simulink model "sm_excv_track1_sprocket"  (R2026a)
settings: Solver=ode23t  StopTime=15  FixedStep=2e-4  AbsTol=1e-3
StartFcn:
  | tic
StopFcn:
  | Elapsed_Sim_Time = toc;
  | disp(['Elapsed Sim Time = ' num2str(Elapsed_Sim_Time)]);
undefined symbols (not defined in the file or in its folder): Excv, X, Y, Z
libraries: sm_lib x11, fl_lib x2, nesl_utility x2, sm_trackV_lib_chain_contact_s46 x2, sm_trackV_lib_chain_underc_elem x1, simulink x1, sm_trackV_lib_chain_contact_s46r9 x1, sm_trackV_lib_chain_track_s46 x1, sm_trackV_lib_chain_underc_i1u2l7 x1
CloseFcn:
  | try,close(h1_sm_excv_track_sprocket),end
  | clear h1_sm_excv_track_sprocket
  | try,close(h2_sm_excv_track_sprocket),end
  | clear h2_sm_excv_track_sprocket
  | try,close(h3_sm_excv_track_sprocket),end
  | clear h3_sm_excv_track_sprocket
  | try,close(h4_sm_excv_track_sprocket),end
  | clear h4_sm_excv_track_sprocket
  | 
  | 
  | clear simlog_sm_excv_track_single_sprocket
  | clear logsout_sm_excv_track_single_sprocket
Description:
  | Excavator Track (Single) Hanging on Sprocket
  | Copyright 2023-2026 The MathWorks, Inc.
settings Model: Creator=evo  LastModifiedBy=smiller
settings SolverCC: ExtrapolationOrder=1.0
settings DataIOCC: SignalLoggingName=logsout_sm_excv_track1_sprocket
settings DebuggingCC: SymbolicDimsDataTypeCodeGenerationDiagnostic=none
settings SimscapeCC: SimscapeNominalValues="[{\"value\":\"1\",\"unit\":\"A\"},{\"value\":\"1\",\"unit\":\"bar\"},{\"value\":\"1\",\"unit\":\"cm^2\"},{\"value\":\"1\",\"unit\":\"cm^3/s\"},{\"value\":\"1\",\"unit\":\"kJ/kg\"},{\"value\":\"1\",\"unit\":\"kW\"},{\"value\":\"1\",\"unit\":\"l\"},{\"value\":\"1\",\"unit\":\"N\"},{\"value\":\"1\",\"unit\":\"N*m\"},{\"value\":\"1\",\"unit\":\"V\"}]"  SimscapeLogSimulationStatistics=on  SimscapeLogName=simlog_sm_excv_track1_sprocket  SimscapeLogLimitData=off
settings DiagnosticsConfigSet: SimMechanicsConflictingReferenceFrames=none
settings ExplorerConfigSet: InternalSimMechanicsExplorerSettings="<ExplorerConfiguration><canonicalview>default</canonicalview><AnimationSetting><BasePlaybackSpeed>1.0</BasePlaybackSpeed><PlaybackSpeedFactor>1.0</PlaybackSpeedFactor></AnimationSetting><TilePanel><TileInfo><Tiles Columns=\"1\" Count=\"1\" Rows=\"1\"><Column Weight=\"1\"/><Row Weight=\"1\"/><Tile Height=\"1\" Width=\"1\" X=\"0\" Y=\"0\"/></Tiles></TileInfo><SceneInfo><SceneViewer><BGColor><R>1</R><G>1</G><B>1</B></BGColor><Camera><DoPerspective>off</DoPerspective><Position><X>-8.59833966249112791e-08</X><Y>-1.5052729587084539</Y><Z>-1.88886838203652996</Z></Position><Center><X>-8.59833966249112791e-08</X><Y>1.09999994761235231</Y><Z>-1.88886838203652996</Z></Center><Up><X>0</X><Y>-0</Y><Z>1</Z></Up><ViewLimDist>1</ViewLimDist><YLim>2.41010291099548368</YLim><XLim>4.22052667248343027</XLim></Camera></SceneViewer></SceneInfo></TilePanel><MechEditorPanel><Cameras/><GfxPanelCameraMap/><VideoCreator><PlaybackSpeedRatio>1.0</PlaybackSpeedRatio><FrameRate>30</FrameRate><VideoFormat>Motion JPEG AVI</VideoFormat><FrameSize>auto</FrameSize></VideoCreator></MechEditorPanel></ExplorerConfiguration>"

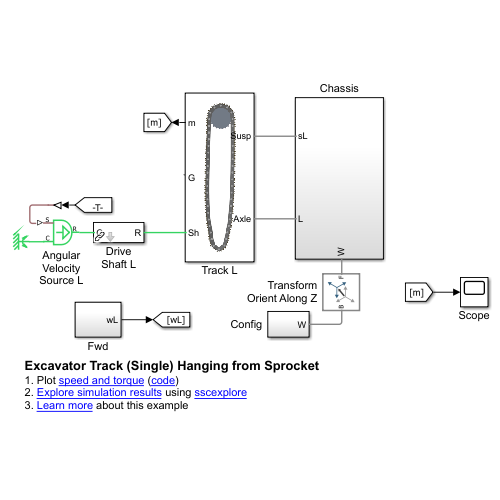
[thumbnail: Simulink's stored preview of the top-level diagram]
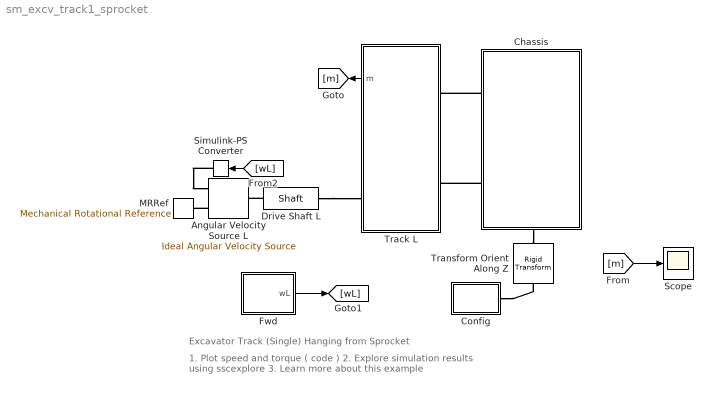
== system sm_excv_track1_sprocket ==
  note: Excavator Track (Single) Hanging from Sprocket
  note: 1. Plot speed and torque ( code )
      | 2. Explore simulation results using sscexplore
      | 3. Learn more about this example
  Angular Velocity Source L : fl_lib/Mechanical/Mechanical Sources/Ideal Angular Velocity Source
  Chassis : Subsystem
      settings: PortSchema="{\"entries\":[{\"content\":{\"sides\":[{\"content\":{\"connectorIds\":[\"LConn1\",\"LConn2\"]},\"type\":\"ConnectorPlacement.EquallySpacedRectSide\",\"uuid\":\"edd0f9cd-c75d-460e-8747-c453c06c3b51\"},{\"content\":{\"side\":\"RIGHT\"},\"type\":\"ConnectorPlacement.EquallySpacedRectSide\",\"uuid\":\"aac0b74e-f978-42e3-a6a1-4bc72aaab1ab\"},{\"content\":{\"side\":\"TOP\"},\"type\":\"ConnectorPlacement.EquallySpacedRectSide\",\"uuid\":\"f25955ca-c2f5-46fd-b059-2b680dae975d\"},{\"content\":{\"connectorIds\":[\"RConn1\"],\"side\":\"BOTTOM\"},\"type\":\"ConnectorPlacement.EquallySpacedRectSide\",\"uuid\":\"7501e828-daf5-40c9-b971-42e639c94cdf\"}]},\"type\":\"ConnectorPlacement.EquallySpacedConnector\",\"uuid\":\"6826b738-8ce7-493d-aa91-65501067c2e5\"}],\"packageUris\":[\"http://schema.mathworks.com/mf0/Connector/R2020b\"],\"version\":\"1.0\"}"
  Config : Subsystem
  Drive Shaft L : sm_trackV_lib_chain_underc_elem/Shaft  k_shaft=Excv.Drive.Shaft.k  b_shaft=Excv.Drive.Shaft.b
  Fwd : Subsystem  VariantControl=Fwd
  MRRef : fl_lib/Mechanical/Rotational Elements/Mechanical Rotational Reference
  Scope : Scope
      settings: ActiveDisplayYMinimum=-3157.84691  ActiveDisplayYMaximum=5645.58158
  Simulink-PS Converter : nesl_utility/Simulink-PS Converter  PhysicalDomain=network_engine_domain  SubClassName=ps_input  LeftPortType=input  RightPortType=output  PseudoPeriodic=off  Frequencies=[]  NoiseDistribution=none  NoiseParameters=[]  Unit=1  AffineConversion=off  FilteringAndDerivatives=provide  SimscapeFilterOrder=1  InputFilterTimeConstant=0.001  UdotUserProvided=0
  Track L : Subsystem
      settings: LibrarySourceBlock=sm_excv_lower_frame_lib/Undercarriage
      mask Display: image('sm_excv_track_sprocket_IMAGE.png');
  Transform Orient Along Z : sm_lib/Frames and Transforms/Rigid Transform  RotationMethod=StandardAxis  FollAlignAxisA=+X  BaseAlignAxisA=+Y  FollAlignAxisB=+Y  BaseAlignAxisB=+Z  RotationStandardAxis=+Y  RotationAngle=90  RotationAngleUnits=deg  RotationArbitraryAxis=[0 0 1]  RotationSequenceAxes=FollowerAxes  RotationSequence=XYX  RotationSequenceAngles=[0 0 0]  RotationSequenceAnglesUnits=deg  RotationMatrix=[1 0 0; 0 1 0; 0 0 1]  Quaternion=[1 0 0 0]  TranslationMethod=None  TranslationCartesianOffset=[0 0 0]  TranslationCartesianOffsetUnits=m  TranslationStandardAxis=+Z  TranslationStandardOffset=0  TranslationStandardOffsetUnits=m  TranslationROffset=0  TranslationROffsetUnits=m  TranslationThetaOffset=0  TranslationThetaOffsetUnits=deg  TranslationZOffset=0  TranslationZOffsetUnits=m
  wires:
  Track L/1(m) -> [m]
  [m] -> Scope/1
  [wL] -> Simulink-PS Converter/1
  Fwd/1(wL) -> [wL]
  connections:
  Chassis/RConn1 -- Transform Orient Along Z/RConn1
  Chassis/LConn2 -- Track L/LConn2
  Config/LConn1 -- Transform Orient Along Z/LConn1
  Angular Velocity Source L/RConn2 -- MRRef/LConn1
  Simulink-PS Converter/RConn1 -- Angular Velocity Source L/RConn1
  Drive Shaft L/LConn1 -- Angular Velocity Source L/LConn1
  Drive Shaft L/RConn1 -- Track L/RConn2
  Chassis/LConn1 -- Track L/LConn1

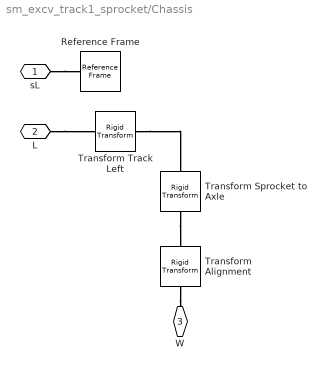
== system sm_excv_track1_sprocket/Chassis ==
  Reference Frame : sm_lib/Frames and Transforms/Reference Frame
  Transform Alignment : sm_lib/Frames and Transforms/Rigid Transform  RotationMethod=AlignedAxes  FollAlignAxisA=+X  BaseAlignAxisA=+X  FollAlignAxisB=+Y  BaseAlignAxisB=+Z  RotationStandardAxis=+Z  RotationAngle=0.0  RotationAngleUnits=deg  RotationArbitraryAxis=[0 0 1]  RotationSequenceAxes=FollowerAxes  RotationSequence=XYX  RotationSequenceAngles=[0 0 0]  RotationSequenceAnglesUnits=deg  RotationMatrix=[1 0 0; 0 1 0; 0 0 1]  Quaternion=[1 0 0 0]  TranslationMethod=None  TranslationCartesianOffset=[0 0 0]  TranslationCartesianOffsetUnits=m  TranslationStandardAxis=+Z  TranslationStandardOffset=0  TranslationStandardOffsetUnits=m  TranslationROffset=0  TranslationROffsetUnits=m  TranslationThetaOffset=0  TranslationThetaOffsetUnits=deg  TranslationZOffset=0  TranslationZOffsetUnits=m
  Transform Sprocket to Axle : sm_lib/Frames and Transforms/Rigid Transform  RotationMethod=None  FollAlignAxisA=+X  BaseAlignAxisA=+Y  FollAlignAxisB=+Y  BaseAlignAxisB=+Z  RotationStandardAxis=+Z  RotationAngle=0.0  RotationAngleUnits=deg  RotationArbitraryAxis=[0 0 1]  RotationSequenceAxes=FollowerAxes  RotationSequence=XYX  RotationSequenceAngles=[0 0 0]  RotationSequenceAnglesUnits=deg  RotationMatrix=[1 0 0; 0 1 0; 0 0 1]  Quaternion=[1 0 0 0]  TranslationMethod=Cartesian  TranslationCartesianOffset=[Excv.Frame.AxleX -Excv.Frame.AxleY 0]  TranslationCartesianOffsetUnits=m  TranslationStandardAxis=+Z  TranslationStandardOffset=0  TranslationStandardOffsetUnits=m  TranslationROffset=0  TranslationROffsetUnits=m  TranslationThetaOffset=0  TranslationThetaOffsetUnits=deg  TranslationZOffset=0  TranslationZOffsetUnits=m
  Transform Track Left : sm_lib/Frames and Transforms/Rigid Transform  RotationMethod=None  FollAlignAxisA=+X  BaseAlignAxisA=+Y  FollAlignAxisB=+Y  BaseAlignAxisB=+Z  RotationStandardAxis=+X  RotationAngle=90  RotationAngleUnits=deg  RotationArbitraryAxis=[0 0 1]  RotationSequenceAxes=FollowerAxes  RotationSequence=XYX  RotationSequenceAngles=[0 0 0]  RotationSequenceAnglesUnits=deg  RotationMatrix=[1 0 0; 0 1 0; 0 0 1]  Quaternion=[1 0 0 0]  TranslationMethod=StandardAxis  TranslationCartesianOffset=[-46.4567 43.3071 -1.4567]  TranslationCartesianOffsetUnits=m  TranslationStandardAxis=-Z  TranslationStandardOffset=1.1  TranslationStandardOffsetUnits=m  TranslationROffset=0  TranslationROffsetUnits=m  TranslationThetaOffset=0  TranslationThetaOffsetUnits=deg  TranslationZOffset=0  TranslationZOffsetUnits=m
  sL : PMIOPort  Side=Left
  L : PMIOPort  Port=2  Side=Left
  W : PMIOPort  Port=3  Side=Right
  connections:
  Transform Alignment/LConn1 -- W/RConn1
  Transform Sprocket to Axle/LConn1 -- Transform Alignment/RConn1
  L/RConn1 -- Transform Track Left/RConn1
  Transform Track Left/LConn1 -- Transform Sprocket to Axle/RConn1
  sL/RConn1 -- Reference Frame/RConn1

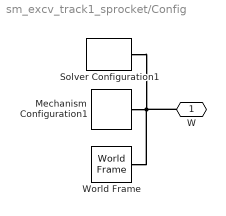
== system sm_excv_track1_sprocket/Config ==
  Mechanism Configuration1 : sm_lib/Utilities/Mechanism Configuration  UniformGravity=Constant  GravityVector=[0 0 -9.80665]  GravityVectorUnits=m/s^2  LinearizationDelta=0.001  JointModeTransitionNonlinearIterations=2
  Solver Configuration1 : nesl_utility/Solver Configuration  PhysicalDomain=network_engine_domain  SubClassName=solver  LeftPortType=input  RightPortType=generic  Tones=[]  Harmonics=[]  SimulateNoise=off  Profile=off  UseLocalSampling=off  EnableSwitchedLinearOptims=on  FrequencyDomain=off  UseCCode=off  RelTol=0.001  AbsTol=0.001  MinStep=1e-09  ToWorkspace=off  RevertToSquareIcSolve=off  NumHomotopyIterations=100  PhasorMode=off  PhasorModeNumHarmonics=1  ConsistencySolver=NEWTON_FTOL  CanonicalOrdering=UNORDERED  OptimizeIntermediates=UNOPTIMIZED  IndexReductionMethod=DerivativeReplacement  DoDC=off  ResidualTolerance=1e-09  ConsistencyTolSource=GLOBAL  ConsistencyAbsTol=0.001  ConsistencyRelTol=0.001  ConsistencyTolFactor=0.001  UseLocalSolver=off  LocalSolverChoice=NE_BACKWARD_EULER_ADVANCER  ResolveIndetEquations=on  FunctionEvalNumThread=1  LocalSolverSampleTime=0.001  DoFixedCost=off  MaxNonlinIter=3  MaxModeIter=2  ComputeImpulses=off  ImpulseIterations=2  LinearAlgebra=auto  LinearAlgebraNumThread=0  EquationFormulation=NE_TIME_EF  DelaysMemoryBudget=1024  AutomaticFiltering=on  FilteringTimeConstant=0.001  PartitionStorageMethod=AS_NEEDED  PartitionMemoryBudget=1024  PartitionMethod=ROBUST  MultibodyUseLocalSolver=off  MultibodyLocalSolverChoice=ODE1  MultibodyLocalSolverSampleTime=0.001
  World Frame : sm_lib/Frames and Transforms/World Frame
  W : PMIOPort  Side=Left
  connections:
  W/RConn1 -- Solver Configuration1/RConn1 -- Mechanism Configuration1/RConn1 -- World Frame/RConn1

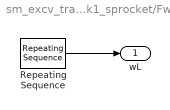
== system sm_excv_track1_sprocket/Fwd ==
  Repeating Sequence : simulink/Sources/Repeating Sequence  rep_seq_t=[0 2 2.01 40]  rep_seq_y=[0 0 3 3]
  wL : Outport
  wires:
  Repeating Sequence/1 -> wL/1

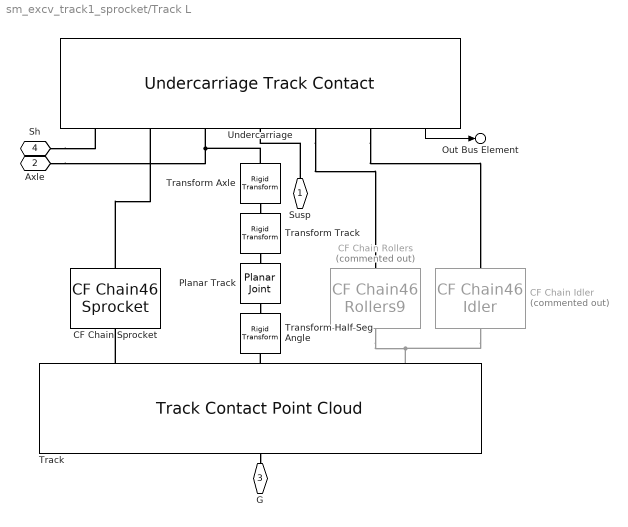
== system sm_excv_track1_sprocket/Track L ==
  CF Chain Idler : sm_trackV_lib_chain_contact_s46/CF Chain46 Idler  Commented=on  K_Idler=Excv.CFP.Idler.K  B_Idler=Excv.CFP.Idler.B  TW_Idler=Excv.CFP.Idler.TW
      settings: LibrarySourceBlock=sm_chain_drive_lib/CF_Idler_full
  CF Chain Rollers : sm_trackV_lib_chain_contact_s46r9/CF Chain46 Rollers9  Commented=on  K_Roller=Excv.Contact.Roller.K  B_Roller=Excv.Contact.Roller.B  TW_Roller=Excv.Contact.Roller.TW
      settings: LibrarySourceBlock=sm_chain_drive_lib/CF Rollers
  CF Chain Sprocket : sm_trackV_lib_chain_contact_s46/CF Chain46 Sprocket  K_Sprocket=Excv.Contact.Sprocket.K  B_Sprocket=Excv.Contact.Sprocket.B  TW_Sprocket=Excv.Contact.Sprocket.TW
      settings: LibrarySourceBlock=sm_chain_drive_lib/CF_Sprocket_full
  Planar Track : sm_lib/Joints/Planar Joint  JointMode=Normal  CompositeWrenchDir=FollowerOnBase  CompositeWrenchFrame=BaseFrame  SenseConstraintForce=off  SenseConstraintTorque=off  SenseTotalForce=off  SenseTotalTorque=off  PxPositionTargetSpecify=off  PxPositionTargetPriority=High  PxPositionTargetValue=0  PxPositionTargetValueUnits=m  PxVelocityTargetSpecify=off  PxVelocityTargetPriority=High  PxVelocityTargetValue=0  PxVelocityTargetValueUnits=m/s  PxEquilibriumPosition=0  PxEquilibriumPositionUnits=m  PxSpringStiffness=0  PxSpringStiffnessUnits=N/m  PxDampingCoefficient=0  PxDampingCoefficientUnits=N/(m/s)  PxLowerLimitSpecify=off  PxLowerLimitBound=-1  PxLowerLimitBoundUnits=m  PxLowerLimitStiffness=1e6  PxLowerLimitStiffnessUnits=N/m  PxLowerLimitDamping=1e3  PxLowerLimitDampingUnits=N/(m/s)  PxLowerLimitTransitionRegionWidth=1e-4  PxLowerLimitTransitionRegionWidthUnits=m  PxUpperLimitSpecify=off  PxUpperLimitBound=1  PxUpperLimitBoundUnits=m  PxUpperLimitStiffness=1e6  PxUpperLimitStiffnessUnits=N/m  PxUpperLimitDamping=1e3  PxUpperLimitDampingUnits=N/(m/s)  PxUpperLimitTransitionRegionWidth=1e-4  PxUpperLimitTransitionRegionWidthUnits=m  PxTorqueActuationMode=NoTorque  PxMotionActuationMode=ComputedMotion  PxSensePosition=off  PxSenseVelocity=off  PxSenseAcceleration=off  PxSenseTorqueForce=off  PxSenseLowerLimitTorqueForce=off  PxSenseUpperLimitTorqueForce=off  PyPositionTargetSpecify=off  PyPositionTargetPriority=High  PyPositionTargetValue=0  PyPositionTargetValueUnits=m  PyVelocityTargetSpecify=off  PyVelocityTargetPriority=High  PyVelocityTargetValue=0  PyVelocityTargetValueUnits=m/s  PyEquilibriumPosition=0  PyEquilibriumPositionUnits=m  PySpringStiffness=0  PySpringStiffnessUnits=N/m  PyDampingCoefficient=0  PyDampingCoefficientUnits=N/(m/s)  PyLowerLimitSpecify=off  PyLowerLimitBound=-1  PyLowerLimitBoundUnits=m  PyLowerLimitStiffness=1e6  PyLowerLimitStiffnessUnits=N/m  PyLowerLimitDamping=1e3  PyLowerLimitDampingUnits=N/(m/s)  PyLowerLimitTransitionRegionWidth=1e-4  PyLowerLimitTransitionRegionWidthUnits=m  PyUpperLimitSpecify=off  PyUpperLimitBound=1  PyUpperLimitBoundUnits=m  PyUpperLimitStiffness=1e6  PyUpperLimitStiffnessUnits=N/m  PyUpperLimitDamping=1e3  PyUpperLimitDampingUnits=N/(m/s)  PyUpperLimitTransitionRegionWidth=1e-4  PyUpperLimitTransitionRegionWidthUnits=m  PyTorqueActuationMode=NoTorque  PyMotionActuationMode=ComputedMotion  PySensePosition=off  PySenseVelocity=off  PySenseAcceleration=off  PySenseTorqueForce=off  PySenseLowerLimitTorqueForce=off  PySenseUpperLimitTorqueForce=off  RzPositionTargetSpecify=on  RzPositionTargetPriority=High  RzPositionTargetValue=0  RzPositionTargetValueUnits=deg  RzVelocityTargetSpecify=off  RzVelocityTargetPriority=High  RzVelocityTargetValue=0  RzVelocityTargetValueUnits=deg/s  RzEquilibriumPosition=0  RzEquilibriumPositionUnits=deg  RzSpringStiffness=0  RzSpringStiffnessUnits=N*m/deg  RzDampingCoefficient=0  RzDampingCoefficientUnits=N*m/(deg/s)  RzLowerLimitSpecify=off  RzLowerLimitBound=-90  RzLowerLimitBoundUnits=deg  RzLowerLimitStiffness=1e4  RzLowerLimitStiffnessUnits=N*m/deg  RzLowerLimitDamping=10  RzLowerLimitDampingUnits=N*m/(deg/s)  RzLowerLimitTransitionRegionWidth=0.1  RzLowerLimitTransitionRegionWidthUnits=deg  RzUpperLimitSpecify=off  RzUpperLimitBound=90  RzUpperLimitBoundUnits=deg  RzUpperLimitStiffness=1e4  RzUpperLimitStiffnessUnits=N*m/deg  RzUpperLimitDamping=10  RzUpperLimitDampingUnits=N*m/(deg/s)  RzUpperLimitTransitionRegionWidth=0.1  RzUpperLimitTransitionRegionWidthUnits=deg  RzTorqueActuationMode=NoTorque  RzMotionActuationMode=ComputedMotion  RzSensePosition=off  RzSenseVelocity=off  RzSenseAcceleration=off  RzSenseTorqueForce=off  RzSenseLowerLimitTorqueForce=off  RzSenseUpperLimitTorqueForce=off
  Track : sm_trackV_lib_chain_track_s46/Track Contact Point Cloud  chain_wid=Excv.Chain.chain_wid  chain_seg_m=Excv.Chain.link_m  chain_seg_cg=Excv.Chain.link_cg  chain_seg_moi=Excv.Chain.link_moi  chain_seg_poi=Excv.Chain.link_poi  plate_h=Excv.Chain.plate_h  plate_xc=Excv.Chain.plate_xc  plate_thk=Excv.Chain.plate_thk  pin_sep=Excv.Chain.pin_sep  plate_ang=Excv.Chain.plate_ang  plate_clr=Excv.Chain.plate_clr  plate_opc=Excv.Chain.plate_opc  pin_len=Excv.Chain.pin_len  pin_rad=Excv.Chain.pin_rad  pin_clr=Excv.Chain.pin_clr  pin_opc=Excv.Chain.pin_opc  shoe_xc=Excv.Shoe.xc  shoe_w=Excv.Shoe.w  shoe_m=Excv.Shoe.mass  shoe_cg=Excv.Shoe.cg  shoe_moi=Excv.Shoe.moi  shoe_poi=Excv.Shoe.poi  shoe_clr=Excv.Shoe.clr  shoe_opc=Excv.Shoe.opc  jointTargets=track_joint_targets  chainDamping=Excv.Chain.damping  ptcld_shoe=Excv.Shoe.ground_contact.ptcld.pts  ptcld_shoe_rad=Excv.Shoe.ground_contact.ptcld.rad  ptcld_shoe_clr=Excv.Shoe.ground_contact.ptcld.clr  ptcld_shoe_opc=Excv.Shoe.ground_contact.ptcld.opc  chain_to_roller_clr=Excv.Chain.roller_contact.clr  chain_to_roller_opc=Excv.Chain.roller_contact.opc  chain_to_teeth_clr=Excv.Chain.teeth_contact.clr  chain_to_teeth_opc=Excv.Chain.teeth_contact.opc
  Transform Axle : sm_lib/Frames and Transforms/Rigid Transform  RotationMethod=None  FollAlignAxisA=+X  BaseAlignAxisA=+Y  FollAlignAxisB=+Y  BaseAlignAxisB=+Z  RotationStandardAxis=+Z  RotationAngle=0.0  RotationAngleUnits=deg  RotationArbitraryAxis=[0 0 1]  RotationSequenceAxes=FollowerAxes  RotationSequence=XYX  RotationSequenceAngles=[0 0 0]  RotationSequenceAnglesUnits=deg  RotationMatrix=[1 0 0; 0 1 0; 0 0 1]  Quaternion=[1 0 0 0]  TranslationMethod=Cartesian  TranslationCartesianOffset=[Excv.Frame.AxleX -Excv.Frame.AxleY 0]  TranslationCartesianOffsetUnits=m  TranslationStandardAxis=+X  TranslationStandardOffset=0  TranslationStandardOffsetUnits=m  TranslationROffset=0  TranslationROffsetUnits=m  TranslationThetaOffset=0  TranslationThetaOffsetUnits=deg  TranslationZOffset=0  TranslationZOffsetUnits=m
  Transform Half Seg Angle : sm_lib/Frames and Transforms/Rigid Transform  RotationMethod=StandardAxis  FollAlignAxisA=+X  BaseAlignAxisA=+Y  FollAlignAxisB=+Y  BaseAlignAxisB=+Z  RotationStandardAxis=+Z  RotationAngle=90-acosd(Excv.Chain.pin_sep/2/Excv.Sprocket.sprocket_rPitch)  RotationAngleUnits=deg  RotationArbitraryAxis=[0 0 1]  RotationSequenceAxes=FollowerAxes  RotationSequence=XYX  RotationSequenceAngles=[0 0 0]  RotationSequenceAnglesUnits=deg  RotationMatrix=[1 0 0; 0 1 0; 0 0 1]  Quaternion=[1 0 0 0]  TranslationMethod=None  TranslationCartesianOffset=[0 0 0]  TranslationCartesianOffsetUnits=m  TranslationStandardAxis=+Z  TranslationStandardOffset=0  TranslationStandardOffsetUnits=m  TranslationROffset=0  TranslationROffsetUnits=m  TranslationThetaOffset=0  TranslationThetaOffsetUnits=deg  TranslationZOffset=0  TranslationZOffsetUnits=m
  Transform Track : sm_lib/Frames and Transforms/Rigid Transform  RotationMethod=StandardAxis  FollAlignAxisA=+X  BaseAlignAxisA=+Y  FollAlignAxisB=+Y  BaseAlignAxisB=+Z  RotationStandardAxis=+Z  RotationAngle=-90  RotationAngleUnits=deg  RotationArbitraryAxis=[0 0 1]  RotationSequenceAxes=FollowerAxes  RotationSequence=XYX  RotationSequenceAngles=[0 0 0]  RotationSequenceAnglesUnits=deg  RotationMatrix=[1 0 0; 0 1 0; 0 0 1]  Quaternion=[1 0 0 0]  TranslationMethod=Cartesian  TranslationCartesianOffset="[-Excv.Sprocket.sprocket_rPitch 0  0]"  TranslationCartesianOffsetUnits=m  TranslationStandardAxis=+Z  TranslationStandardOffset=0  TranslationStandardOffsetUnits=m  TranslationROffset=0  TranslationROffsetUnits=m  TranslationThetaOffset=0  TranslationThetaOffsetUnits=deg  TranslationZOffset=0  TranslationZOffsetUnits=m
  Undercarriage : sm_trackV_lib_chain_underc_i1u2l7/Undercarriage Track Contact  popup_leftOrRight=Left  sprk_xc=Excv.Sprocket.sprocket_xc  sprk_len=Excv.Sprocket.sprk_width  sprk_rho=Excv.Sprocket.density  sprk_clr=Excv.Sprocket.clr  sprk_opc=Excv.Sprocket.opc  sprk_contact_geo_ptcld=Excv.Sprocket.teeth_contact.ptcld.pts  sprk_contact_geo_rad=Excv.Sprocket.teeth_contact.ptcld.rad  sprk_contact_geo_clr=Excv.Sprocket.teeth_contact.ptcld.clr  sprk_contact_geo_opc=Excv.Sprocket.teeth_contact.ptcld.opc  idler_rad=Excv.Idler.rad  idler_len=Excv.Idler.len  idler_rho=Excv.Idler.rho  idler_clr=Excv.Idler.clr  idler_opc=Excv.Idler.opc  idler_contgeo_clr=Excv.Idler.chain_contact.clr  idler_contgeo_opc=Excv.Idler.chain_contact.opc  roller_upper_rad=Excv.Roller.Upper.rad  roller_upper_len=Excv.Roller.Upper.len  roller_upper_rho=Excv.Roller.Upper.rho  roller_upper_clr=Excv.Roller.Upper.clr  roller_upper_opc=Excv.Roller.Upper.opc  roller_upper_contgeo_clr=[1.0 0.0 0.0]  roller_upper_contgeo_opc=1  roller_lower_rad=Excv.Roller.Lower.rad  roller_lower_len=Excv.Roller.Lower.len  roller_lower_rho=Excv.Roller.Lower.rho  roller_lower_clr=Excv.Roller.Lower.clr  roller_lower_opc=Excv.Roller.Lower.opc  roller_lower_contgeo_clr=[1.0 0.0 0.0]  roller_lower_contgeo_opc=1  tensioner_cyl_len=Excv.Idler.Tensioner.cyl.len  tensioner_cyl_rad=Excv.Idler.Tensioner.cyl.rad  tensioner_cyl_rho=Excv.Idler.Tensioner.cyl.rho  tensioner_cyl_clr=Excv.Idler.Tensioner.cyl.clr  tensioner_cyl_opc=Excv.Idler.Tensioner.cyl.opc  tensioner_pist_len=Excv.Idler.Tensioner.piston.len  tensioner_pist_rad=Excv.Idler.Tensioner.piston.rad  tensioner_pist_rho=Excv.Idler.Tensioner.piston.rho  tensioner_pist_clr=Excv.Idler.Tensioner.piston.clr  tensioner_pist_opc=Excv.Idler.Tensioner.piston.opc  tensioner_br_length=Excv.Idler.Tensioner.bracket.len  tensioner_br_width=Excv.Idler.Tensioner.bracket.wid  tensioner_br_height=Excv.Idler.Tensioner.bracket.height  tensioner_br_thk=Excv.Idler.Tensioner.bracket.thk  tensioner_br_rho=Excv.Idler.Tensioner.bracket.rho  tensioner_br_clr=Excv.Idler.Tensioner.bracket.clr  tensioner_br_opc=Excv.Idler.Tensioner.bracket.opc  tensioner_eqpos=Excv.Idler.Tensioner.xeq  tensioner_x0=Excv.Idler.Tensioner.x0  tensioner_k=Excv.Idler.Tensioner.K  tensioner_b=Excv.Idler.Tensioner.B  roller_upper_x=Excv.Frame.Sprk2UpperX  roller_lower_x=Excv.Frame.Sprk2LowerX  idler_x=Excv.Frame.IdlerAssyX  axle_x=Excv.Frame.AxleX  roller_upper_y=Excv.Frame.Sprk2UpperY  roller_lower_y=Excv.Frame.Sprk2LowerY  idler_y=Excv.Frame.Sprk2IdlerY  axle_y=Excv.Frame.AxleY  frame_cg_offset=Excv.Frame.CGOffset  frame_mass=Excv.Frame.Mass  frame_moi=Excv.Frame.MOI  frame_poi=Excv.Frame.POI  frame_susp_offset=Excv.Frame.SuspOffset  popup_sense_roller=Actuator Torque
  Susp : PMIOPort  Side=Left
  Axle : PMIOPort  Port=2  Side=Left
  G : PMIOPort  Port=3  Side=Right
  Sh : PMIOPort  Port=4  Side=Right
  Out Bus Element : Outport  PortName=m  Element=Underc
  wires:
  Undercarriage/1 -> Out Bus Element/1
  connections:
  Track/LConn2 -- Transform Half Seg Angle/RConn1
  Track/LConn3 -- CF Chain Sprocket/RConn1
  Undercarriage/RConn1 -- CF Chain Idler/LConn1
  Undercarriage/RConn2 -- CF Chain Rollers/LConn1
  Track/RConn1 -- G/RConn1
  CF Chain Idler/RConn1 -- Track/LConn1 -- CF Chain Rollers/RConn1
  Transform Track/RConn1 -- Planar Track/LConn1
  Planar Track/RConn1 -- Transform Half Seg Angle/LConn1
  Sh/RConn1 -- Undercarriage/RConn6
  CF Chain Sprocket/LConn1 -- Undercarriage/RConn5
  Transform Axle/LConn1 -- Transform Track/LConn1
  Transform Axle/RConn1 -- Axle/RConn1 -- Undercarriage/RConn4
  Susp/RConn1 -- Undercarriage/RConn3
